simulink model "NBMSState"  (R2024b)
settings: configuration reference "STM32H7_Config" (kept outside this file)
settings Model: DataDictionary=Master_Dictionary.sldd  EnableAccessToBaseWorkspace=off  Creator=torni  LastModifiedBy=William
settings ConfigSetRef: SourceName=STM32H7_Config

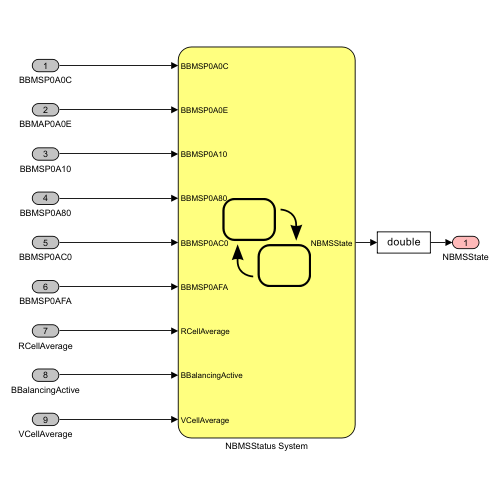
[thumbnail: Simulink's stored preview of the top-level diagram]
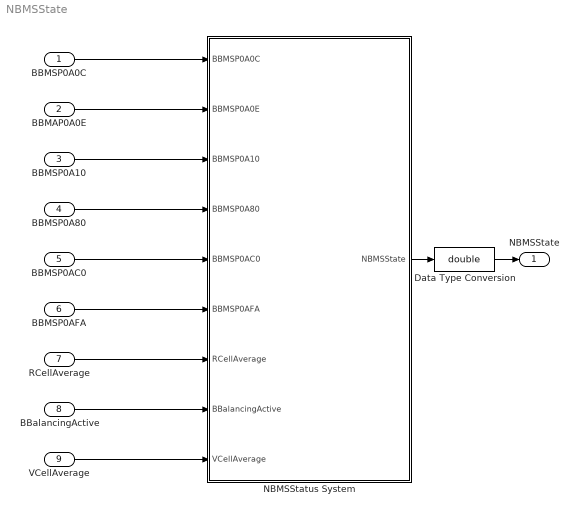
== system NBMSState ==
  BBMSP0A0C : Inport  OutDataTypeStr=boolean
  BBMAP0A0E : Inport  Port=2  OutDataTypeStr=boolean
  BBMSP0A10 : Inport  Port=3  OutDataTypeStr=boolean
  BBMSP0A80 : Inport  Port=4  OutDataTypeStr=boolean
  BBMSP0AC0 : Inport  Port=5  OutDataTypeStr=boolean
  BBMSP0AFA : Inport  Port=6  OutDataTypeStr=boolean
  RCellAverage : Inport  Port=7  OutDataTypeStr=double
  BBalancingActive : Inport  Port=8  OutDataTypeStr=boolean
  VCellAverage : Inport  Port=9  OutDataTypeStr=double
  Data Type Conversion : DataTypeConversion  OutDataTypeStr=double  SaturateOnIntegerOverflow=off  RndMeth=Floor
  NBMSStatus System : Stateflow chart  TreatAsAtomicUnit=on
  NBMSState : Outport  OutDataTypeStr=double  VectorParamsAs1DForOutWhenUnconnected=off
  wires:
  BBalancingActive/1 -> NBMSStatus System/8(BBalancingActive)
  RCellAverage/1 -> NBMSStatus System/7(RCellAverage)
  BBMSP0AC0/1 -> NBMSStatus System/5(BBMSP0AC0)
  BBMAP0A0E/1 -> NBMSStatus System/2(BBMSP0A0E)
  BBMSP0AFA/1 -> NBMSStatus System/6(BBMSP0AFA)
  BBMSP0A10/1 -> NBMSStatus System/3(BBMSP0A10)
  BBMSP0A0C/1 -> NBMSStatus System/1(BBMSP0A0C)
  BBMSP0A80/1 -> NBMSStatus System/4(BBMSP0A80)
  VCellAverage/1 -> NBMSStatus System/9(VCellAverage)
  NBMSStatus System/1(NBMSState) -> Data Type Conversion/1
  Data Type Conversion/1 -> NBMSState/1

== stateflow chart NBMSState/NBMSStatus System ==
  state BMSError = BBMSError [function]
    note: Highest cell voltage too high - P0A0C
        | Lowest cell voltage too low - P0A0E
        | Pack too hot fault - P0A10
        | Weak cell fault - P0A80
        | Current sensor fault - P0AC0
        | Low cell voltage fault - P0AFA
    (default) -> (junction 116) : {BMSError = 0}
    (junction 116) -> (junction 118) : [BBalancingActive==1 ||...
        | RCellAverage<0 ||...
        | VCellAverage<0 ||...
        | BBMSP0A0C==1 ||...
        | BBMSP0A0E==1 ||...
        | BBMSP0A10==1 ||...
        | BBMSP0A80==1 ||...
        | BBMSP0AC0==1||...
        | BBMSP0AFA==1]
    (junction 118) -> (junction 121) : {BMSError = 1}
  state BMS_States [group]
    state Idle
      entry:
      NBMSState = 0
    state State_9
      entry:
      NBMSState = 9
    state State_1
      entry:
      NBMSState = 1
    state State_2
      entry:
      NBMSState = 2
    state State_8
      entry:
      NBMSState = 8
    state State_3
      entry:
      NBMSState = 3
    state State_7
      entry:
      NBMSState = 7
    state State_4
      entry:
      NBMSState = 4
    state State_6
      entry:
      NBMSState = 6
    state State_5
      entry:
      NBMSState = 5
    (default) -> Idle
    Idle -> State_1 : after (7000, tick)
    State_8 -> State_9 [order 2] : [BBMSP0AC0==0]
    State_1 -> State_2 [order 2] : [BBalancingActive==0]
    (junction 67) -> State_1
    State_9 -> (junction 67) [order 2] : [BBMSError()==1]
    State_1 -> (junction 67) [order 1] : [BBMSError()==1]
    State_2 -> (junction 67) [order 1] : [BBMSError()==1]
    State_8 -> (junction 67) [order 1] : [BBMSError()==1]
    State_2 -> State_3 [order 2] : [RCellAverage >= 0]
    State_7 -> State_8 [order 2] : [BBMSP0A80==0]
    State_7 -> (junction 67) [order 1] : [BBMSError()==1]
    State_3 -> (junction 67) [order 1] : [BBMSError()==1]
    State_6 -> (junction 67) [order 1] : [BBMSError()==1]
    State_4 -> (junction 67) [order 1] : [BBMSError()==1]
    State_5 -> (junction 67) [order 1] : [BBMSError()==1]
    State_3 -> State_4 [order 2] : [VCellAverage>=0]
    State_6 -> State_7 [order 2] : [BBMSP0A10==0]
    State_4 -> State_5 [order 2] : [BBMSP0A0C==0]
    State_5 -> State_6 [order 2] : [BBMSP0A0E==0]
  state BMS_OK
    entry:
    NBMSState = 92
  BMS_OK -> (junction 67) : [BBMSError()==1]
  State_9 -> BMS_OK [order 1] : [BBMSP0AFA==0]
  data: BMSError function_output double; BBMSP0A0C input boolean; BBMSP0A0E input boolean; BBMSP0A10 input boolean; BBMSP0A80 input boolean; BBMSP0AC0 input boolean; BBMSP0AFA input boolean; RCellAverage input double; BBalancingActive input boolean; VCellAverage input double; NBMSState output double
